simulink model "ricatti"  (R2021b)
settings: Solver=VariableStepAuto  StartTime=0.0  StopTime=20  RelTol=1e-3
values from neighbouring files (symbols this model uses):
  A = [0 w_0(3) -w_0(2) 0 x_0(3) -x_0(2) ... (first row only)    [kalman_ex_5.m]    (also in pitch_kalman.m = 0; pitch_kalman_bias.m = [0 -1;0 0]; roll_kalman.m = 0; roll_kalman_bias.m = [0 -1;0 0])
  C = [eye(3) zeros(3,3)]    [kalman_ex_5.m]    (also in pitch_kalman.m = 1; pitch_kalman_bias.m = [1 0]; roll_kalman.m = 1; roll_kalman_bias.m = [1 0])
  Q = diag([100*cov_wx 100*cov_wy 100*cov_wz 0.1*cov_wx 0.1*cov_wy 0.1*cov_wz])    [kalman_ex_5.m]    (also in pitch_kalman.m = cov_wy; pitch_kalman_bias.m = diag([10000*cov_wy cov_wy]); roll_kalman.m = cov_wx; roll_kalman_bias.m = diag([10000*cov_wx cov_wx]))
  R = 100*R    [kalman_ex_5.m]    (also in pitch_kalman.m = 10*cov_pitch_acel; pitch_kalman_bias.m = 10*cov_pitch_acel; roll_kalman.m = 10*cov_roll_acel; roll_kalman_bias.m = 10*cov_roll_acel)
settings Model: Creator=sasas  LastModifiedBy=p28ma
settings SolverCC: AlgebraicLoopSolver=TrustRegion
settings DebuggingCC: SFMachineParentedDataDiag=warning

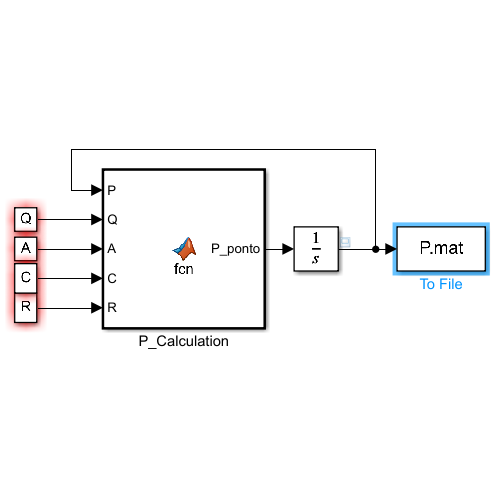
[thumbnail: Simulink's stored preview of the top-level diagram]
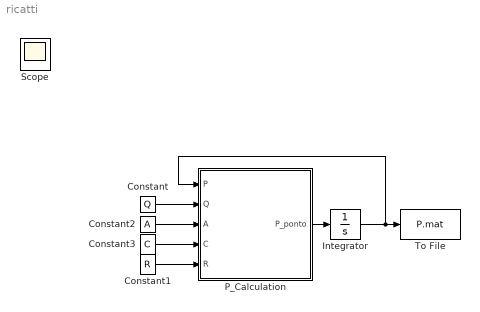
== system ricatti ==
  Constant : Constant  Value=Q
  Constant1 : Constant  Value=R
  Constant2 : Constant  Value=A
  Constant3 : Constant  Value=C
  Integrator : Integrator
  P_Calculation : MATLAB Function  TreatAsAtomicUnit=on
  To File : ToFile  Filename=P.mat  MatrixName=P  SaveFormat=Timeseries
  Scope : Scope
  wires:
  P_Calculation/1(P_ponto) -> Integrator/1
  Constant/1 -> P_Calculation/2(Q)
  Constant1/1 -> P_Calculation/5(R)
  Integrator/1 -> P_Calculation/1(P), To File/1
  Constant2/1 -> P_Calculation/3(A)
  Constant3/1 -> P_Calculation/4(C)

== matlab function ricatti/P_Calculation ==
  data: P input; P_ponto output; Q input; A input; C input; R input
function P_ponto = fcn(P,Q,A,C,R)
P_ponto = A*P+P*A'+Q-P*C'*inv(R)*C*P;
